simulink library "vehdynlibtire_TUM"  (R2018b)
settings: Solver=ode45  StartTime=0.0  StopTime=10.0  RelTol=1e-3  EnableMultiTasking=on
libraries: vehdynlibtirecommon x2, vehdynlibtirecommon_TUM x1
(part 2 of 2)

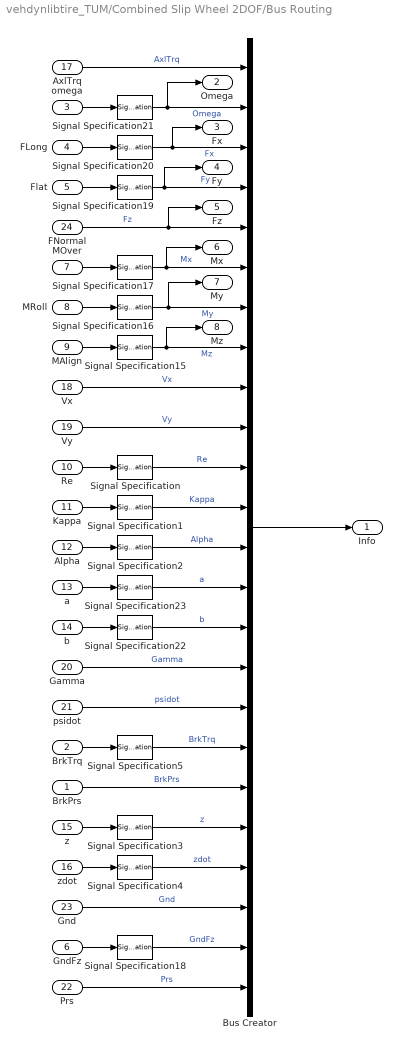
== system vehdynlibtire_TUM/Combined Slip Wheel 2DOF/Bus Routing ==
  BrkPrs : Inport
  BrkTrq : Inport  Port=2
  omega : Inport  Port=3
  FLong : Inport  Port=4
  Flat : Inport  Port=5
  GndFz : Inport  Port=6
  MOver : Inport  Port=7
  MRoll : Inport  Port=8
  MAlign : Inport  Port=9
  Re : Inport  Port=10
  Kappa : Inport  Port=11
  Alpha : Inport  Port=12
  a : Inport  Port=13
  b : Inport  Port=14
  z : Inport  Port=15
  zdot : Inport  Port=16
  AxlTrq : Inport  Port=17
  Vx : Inport  Port=18
  Vy : Inport  Port=19
  Gamma : Inport  Port=20
  psidot : Inport  Port=21
  Prs : Inport  Port=22
  Gnd : Inport  Port=23
  FNormal : Inport  Port=24
  Bus Creator : BusCreator  Inputs=24
  Signal Specification{,3,22..23} (4 alike) : SignalSpecification  Unit=m
  Signal Specification1 : SignalSpecification  Unit=1
  Signal Specification{5,15..17} (4 alike) : SignalSpecification  Unit=N*m
  Signal Specification18 : SignalSpecification  Unit=N
  Signal Specification19 : SignalSpecification  Unit=N
  Signal Specification2 : SignalSpecification  Unit=rad
  Signal Specification20 : SignalSpecification  Unit=N
  Signal Specification21 : SignalSpecification  Unit=rad/s
  Signal Specification4 : SignalSpecification  Unit=m/s
  Info : Outport
  Omega : Outport  Port=2  Unit=rad/s
  Fx : Outport  Port=3  Unit=N
  Fy : Outport  Port=4  Unit=N
  Fz : Outport  Port=5  Unit=N
  Mx : Outport  Port=6  Unit=N*m
  My : Outport  Port=7  Unit=N*m
  Mz : Outport  Port=8  Unit=N*m
  wires:
  Signal Specification3/1 -> Bus Creator/20  "z"
  a/1 -> Signal Specification23/1
  Alpha/1 -> Signal Specification2/1
  Signal Specification4/1 -> Bus Creator/21  "zdot"
  Signal Specification21/1 -> Bus Creator/2, Omega/1  "Omega"
  FNormal/1 -> Bus Creator/5, Fz/1  "Fz"
  Signal Specification15/1 -> Bus Creator/8, Mz/1  "Mz"
  Signal Specification/1 -> Bus Creator/11  "Re"
  Bus Creator/1 -> Info/1
  Signal Specification17/1 -> Mx/1, Bus Creator/6  "Mx"
  MOver/1 -> Signal Specification17/1
  Signal Specification1/1 -> Bus Creator/12  "Kappa"
  FLong/1 -> Signal Specification20/1
  Signal Specification19/1 -> Bus Creator/4, Fy/1  "Fy"
  Signal Specification16/1 -> Bus Creator/7, My/1  "My"
  omega/1 -> Signal Specification21/1
  Signal Specification2/1 -> Bus Creator/13  "Alpha"
  Signal Specification20/1 -> Bus Creator/3, Fx/1  "Fx"
  Signal Specification23/1 -> Bus Creator/14  "a"
  Signal Specification22/1 -> Bus Creator/15  "b"
  GndFz/1 -> Signal Specification18/1
  MAlign/1 -> Signal Specification15/1
  Flat/1 -> Signal Specification19/1
  b/1 -> Signal Specification22/1
  Re/1 -> Signal Specification/1
  zdot/1 -> Signal Specification4/1
  z/1 -> Signal Specification3/1
  MRoll/1 -> Signal Specification16/1
  Kappa/1 -> Signal Specification1/1
  BrkTrq/1 -> Signal Specification5/1
  AxlTrq/1 -> Bus Creator/1  "AxlTrq"
  Vx/1 -> Bus Creator/9  "Vx"
  Vy/1 -> Bus Creator/10  "Vy"
  Gamma/1 -> Bus Creator/16  "Gamma"
  psidot/1 -> Bus Creator/17  "psidot"
  Signal Specification5/1 -> Bus Creator/18  "BrkTrq"
  BrkPrs/1 -> Bus Creator/19  "BrkPrs"
  Signal Specification18/1 -> Bus Creator/23  "GndFz"
  Gnd/1 -> Bus Creator/22  "Gnd"
  Prs/1 -> Bus Creator/24  "Prs"

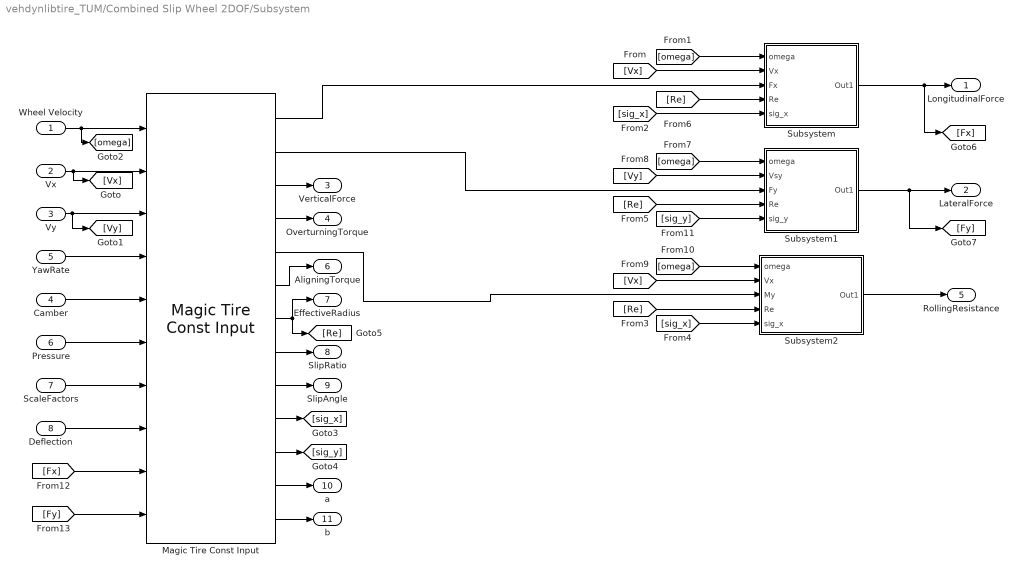
== system vehdynlibtire_TUM/Combined Slip Wheel 2DOF/Subsystem ==
  Wheel Velocity : Inport
  Vx : Inport  Port=2
  Vy : Inport  Port=3
  Camber : Inport  Port=4
  YawRate : Inport  Port=5
  Pressure : Inport  Port=6
  ScaleFactors : Inport  Port=7
  Deflection : Inport  Port=8
  Magic Tire Const Input : vehdynlibtirecommon_TUM/Magic Tire Const Input/Magic Tire Const Input  SystemSampleTime=-1
  Subsystem : Subsystem
  Subsystem1 : Subsystem
  Subsystem2 : Subsystem
  LongitudinalForce : Outport
  LateralForce : Outport  Port=2
  VerticalForce : Outport  Port=3
  OverturningTorque : Outport  Port=4
  RollingResistance : Outport  Port=5
  AligningTorque : Outport  Port=6
  EffectiveRadius : Outport  Port=7
  SlipRatio : Outport  Port=8
  SlipAngle : Outport  Port=9
  a : Outport  Port=10
  b : Outport  Port=11
  wires:
  [Re] -> Subsystem/4(Re)
  Magic Tire Const Input/11 -> [sig_y]
  Magic Tire Const Input/9 -> SlipAngle/1
  Magic Tire Const Input/6 -> AligningTorque/1
  [omega] -> Subsystem2/1(omega)
  Magic Tire Const Input/13 -> b/1
  [sig_x] -> Subsystem2/5(sig_x)
  [Vy] -> Subsystem1/2(Vsy)
  [Vx] -> Subsystem2/2(Vx)
  [Re] -> Subsystem2/4(Re)
  [Fx] -> Magic Tire Const Input/9
  Pressure/1 -> Magic Tire Const Input/6
  [Fy] -> Magic Tire Const Input/10
  Subsystem2/1(Out1) -> RollingResistance/1
  Vy/1 -> [Vy], Magic Tire Const Input/3
  Deflection/1 -> Magic Tire Const Input/8
  [sig_y] -> Subsystem1/5(sig_y)
  Magic Tire Const Input/7 -> [Re], EffectiveRadius/1
  ScaleFactors/1 -> Magic Tire Const Input/7
  Magic Tire Const Input/8 -> SlipRatio/1
  Vx/1 -> [Vx], Magic Tire Const Input/2
  Wheel Velocity/1 -> Magic Tire Const Input/1, [omega]
  Camber/1 -> Magic Tire Const Input/5
  Magic Tire Const Input/12 -> a/1
  Magic Tire Const Input/10 -> [sig_x]
  Subsystem1/1(Out1) -> LateralForce/1, [Fy]
  [Re] -> Subsystem1/4(Re)
  Magic Tire Const Input/2 -> Subsystem1/3(Fy)
  Magic Tire Const Input/4 -> OverturningTorque/1
  Subsystem/1(Out1) -> [Fx], LongitudinalForce/1
  [omega] -> Subsystem1/1(omega)
  [Vx] -> Subsystem/2(Vx)
  Magic Tire Const Input/3 -> VerticalForce/1
  YawRate/1 -> Magic Tire Const Input/4
  [omega] -> Subsystem/1(omega)
  [sig_x] -> Subsystem/5(sig_x)
  Magic Tire Const Input/5 -> Subsystem2/3(My)
  Magic Tire Const Input/1 -> Subsystem/3(Fx)

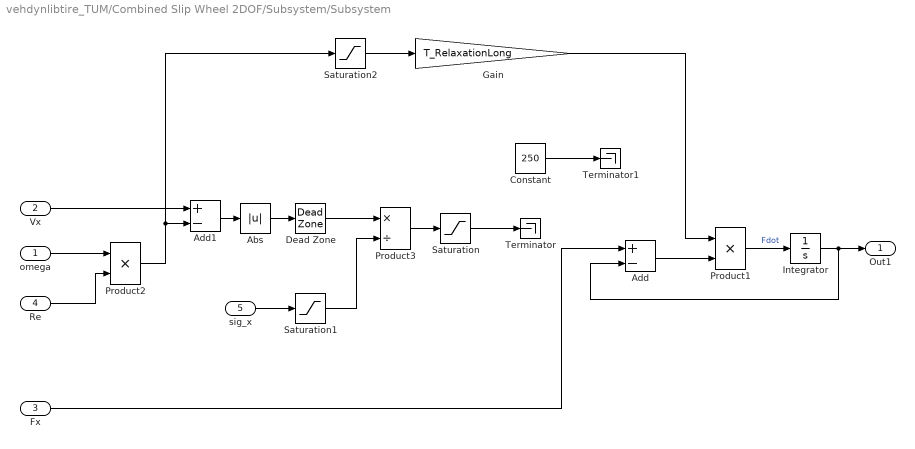
== system vehdynlibtire_TUM/Combined Slip Wheel 2DOF/Subsystem/Subsystem ==
  omega : Inport
  Vx : Inport  Port=2
  Fx : Inport  Port=3
  Re : Inport  Port=4
  sig_x : Inport  Port=5
  Abs : Abs  ZeroCross=off
  Add : Sum  Inputs=+-
  Add1 : Sum  Inputs=+-
  Constant : Constant  Value=250
  Dead Zone : DeadZone  LowerValue=0  UpperValue=VXLOW  ZeroCross=off  SaturateOnIntegerOverflow=on
  Gain : Gain  Gain=T_RelaxationLong
  Integrator : Integrator  UpperSaturationLimit=10e3  LowerSaturationLimit=-10e3  AbsoluteTolerance=1e-3  ZeroCross=off
  Product1 : Product  Inputs=**
  Product2 : Product  Inputs=**
  Product3 : Product  Inputs=*/
  Saturation : Saturate  UpperLimit=400*pi*2  LowerLimit=2*pi  ZeroCross=off
  Saturation1 : Saturate  UpperLimit=10  LowerLimit=.01  ZeroCross=off
  Saturation2 : Saturate  UpperLimit=100  LowerLimit=10
  Terminator : Terminator
  Terminator1 : Terminator
  Out1 : Outport  PortDimensions=1
  wires:
  Gain/1 -> Product1/1
  sig_x/1 -> Saturation1/1
  Saturation1/1 -> Product3/2
  Product1/1 -> Integrator/1  "Fdot"
  Dead Zone/1 -> Product3/1
  Constant/1 -> Terminator1/1
  Saturation/1 -> Terminator/1
  Fx/1 -> Add/1
  Integrator/1 -> Add/2, Out1/1
  Abs/1 -> Dead Zone/1
  Product3/1 -> Saturation/1
  Vx/1 -> Add1/1
  Product2/1 -> Saturation2/1, Add1/2
  Saturation2/1 -> Gain/1
  Re/1 -> Product2/2
  Add/1 -> Product1/2
  Add1/1 -> Abs/1
  omega/1 -> Product2/1

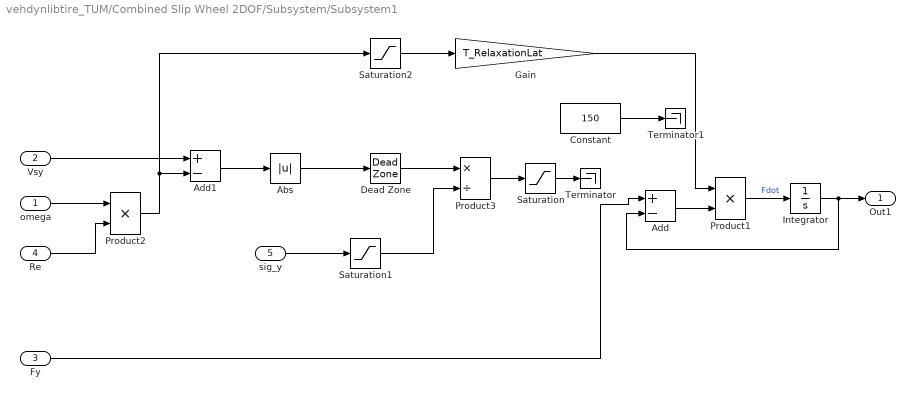
== system vehdynlibtire_TUM/Combined Slip Wheel 2DOF/Subsystem/Subsystem1 ==
  omega : Inport
  Vsy : Inport  Port=2
  Fy : Inport  Port=3
  Re : Inport  Port=4
  sig_y : Inport  Port=5
  Abs : Abs  ZeroCross=off
  Add : Sum  Inputs=+-
  Add1 : Sum  Inputs=+-
  Constant : Constant  Value=150
  Dead Zone : DeadZone  LowerValue=0  UpperValue=VXLOW  ZeroCross=off  SaturateOnIntegerOverflow=on
  Gain : Gain  Gain=T_RelaxationLat
  Integrator : Integrator  UpperSaturationLimit=10e3  LowerSaturationLimit=-10e3  AbsoluteTolerance=1e-3  ZeroCross=off
  Product1 : Product  Inputs=**
  Product2 : Product  Inputs=**
  Product3 : Product  Inputs=*/
  Saturation : Saturate  UpperLimit=400*pi  LowerLimit=2*pi  ZeroCross=off
  Saturation1 : Saturate  UpperLimit=10  LowerLimit=.01  ZeroCross=off
  Saturation2 : Saturate  UpperLimit=100  LowerLimit=1
  Terminator : Terminator
  Terminator1 : Terminator
  Out1 : Outport  PortDimensions=1
  wires:
  Integrator/1 -> Out1/1, Add/2
  Gain/1 -> Product1/1
  Saturation2/1 -> Gain/1
  Constant/1 -> Terminator1/1
  Product3/1 -> Saturation/1
  Abs/1 -> Dead Zone/1
  sig_y/1 -> Saturation1/1
  Dead Zone/1 -> Product3/1
  Saturation1/1 -> Product3/2
  Add1/1 -> Abs/1
  Saturation/1 -> Terminator/1
  Add/1 -> Product1/2
  omega/1 -> Product2/1
  Re/1 -> Product2/2
  Product2/1 -> Saturation2/1, Add1/2
  Vsy/1 -> Add1/1
  Product1/1 -> Integrator/1  "Fdot"
  Fy/1 -> Add/1

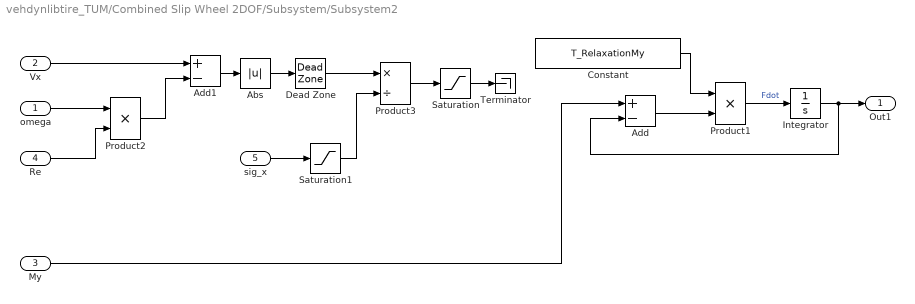
== system vehdynlibtire_TUM/Combined Slip Wheel 2DOF/Subsystem/Subsystem2 ==
  omega : Inport
  Vx : Inport  Port=2
  My : Inport  Port=3
  Re : Inport  Port=4
  sig_x : Inport  Port=5
  Abs : Abs  ZeroCross=off
  Add : Sum  Inputs=+-
  Add1 : Sum  Inputs=+-
  Constant : Constant  Value=T_RelaxationMy
  Dead Zone : DeadZone  LowerValue=0  UpperValue=VXLOW  ZeroCross=off  SaturateOnIntegerOverflow=on
  Integrator : Integrator  UpperSaturationLimit=10e3  LowerSaturationLimit=-10e3  AbsoluteTolerance=1e-3  ZeroCross=off
  Product1 : Product  Inputs=**
  Product2 : Product  Inputs=**
  Product3 : Product  Inputs=*/
  Saturation : Saturate  UpperLimit=400*pi*2  LowerLimit=2*pi  ZeroCross=off
  Saturation1 : Saturate  UpperLimit=10  LowerLimit=.01  ZeroCross=off
  Terminator : Terminator
  Out1 : Outport  PortDimensions=1
  wires:
  Abs/1 -> Dead Zone/1
  Saturation/1 -> Terminator/1
  Saturation1/1 -> Product3/2
  Constant/1 -> Product1/1
  My/1 -> Add/1
  Vx/1 -> Add1/1
  Add1/1 -> Abs/1
  Product2/1 -> Add1/2
  Product3/1 -> Saturation/1
  Add/1 -> Product1/2
  Integrator/1 -> Out1/1, Add/2
  sig_x/1 -> Saturation1/1
  Product1/1 -> Integrator/1  "Fdot"
  Re/1 -> Product2/2
  Dead Zone/1 -> Product3/1
  omega/1 -> Product2/1
